simulink model "Controller_PP_test"  (R2021a)
settings: Solver=FixedStepDiscrete  StartTime=0.0  StopTime=inf  FixedStep=0.05  RelTol=1e-3
PostLoadFcn:
  | , if any(exist('dsrtsu_mdlpostloadfcn', 'file') == [2, 3, 6]), try dsrtsu_mdlpostloadfcn('Execute', bdroot); catch fprintf('Error in PostLoadFcn (dsrtsu_mdlpostloadfcn) for model "%s":\n %s\n', bdroot, lasterr); end, end,
model workspace (MAT data in the model file):
  DLC_kr = [-5.84862481044e-05 -6.43095507895e-05 -7.01328534794e-05 -7.5956156174e-05 -8.17794588731e-05 -8.76027615758e-05 -9.34260642811e-05 -9.92493669872e-05 -0.000105072669692 -0.000110895972393 -0.000116719275087 -0.000122542545808 ... (2080 elements, 1x2080)]
  DLC_thetar = [1.57172954906 1.57172588114 1.57172186534 1.57171750165 1.57171279008 1.57170773062 1.57170232328 1.57169656806 1.57169046495 1.57168401395 1.57167721507 1.57167006831 ... (2080 elements, 1x2080)]
  DLC_xr = [-0.00056695162723 -0.000622594591628 -0.000678008043004 -0.000733171198692 -0.000788063276025 -0.000842663492338 -0.000896951064963 -0.000950905211235 -0.00100450514849 -0.00105773009405 -0.00111055926527 -0.00116297187948 ... (2080 elements, 1x2080)]
  DLC_yr = [0.59999973213 0.659739817002 0.719479902091 0.779219987412 0.838960072984 0.898700158824 0.958440244948 1.01818033138 1.07792041812 1.1376605052 1.19740059264 1.25714068045 ... (2080 elements, 1x2080)]
  Fliter_ = 0.5
  Fliter_k = 1
  Iz = 1650
  SL_ROS_VariableLengthArrays_MaxSizes.CommonInfo.ArrayTruncateAction = 'EmitWarning'
  SL_ROS_VariableLengthArrays_MaxSizes.MsgTypeMap = containers.Map
  SL_ROS_VariableLengthArrays_MaxSizes.MsgTypeMap.serialization.keys = {'std_msgs/Float32MultiArray', 'std_msgs/Float64MultiArray', 'std_msgs/Int16MultiArray'}
  SL_ROS_VariableLengthArrays_MaxSizes.MsgTypeMap.serialization.values{1}.PropertyName = 'Data'
  SL_ROS_VariableLengthArrays_MaxSizes.MsgTypeMap.serialization.values{1}.DataType = 'single'
  SL_ROS_VariableLengthArrays_MaxSizes.MsgTypeMap.serialization.values{1}.MaxLength = 2004
  SL_ROS_VariableLengthArrays_MaxSizes.MsgTypeMap.serialization.values{2}.PropertyName = 'Data'
  SL_ROS_VariableLengthArrays_MaxSizes.MsgTypeMap.serialization.values{2}.DataType = 'double'
  SL_ROS_VariableLengthArrays_MaxSizes.MsgTypeMap.serialization.values{2}.MaxLength = 3
  SL_ROS_VariableLengthArrays_MaxSizes.MsgTypeMap.serialization.values{3}.PropertyName = 'Data'
  SL_ROS_VariableLengthArrays_MaxSizes.MsgTypeMap.serialization.values{3}.DataType = 'int16'
  SL_ROS_VariableLengthArrays_MaxSizes.MsgTypeMap.serialization.values{3}.MaxLength = 5
  SL_ROS_VariableLengthArrays_MaxSizes.MsgTypeMap.serialization.uniformity = 0
  SL_ROS_VariableLengthArrays_MaxSizes.MsgTypeMap.serialization.keyType = 'char'
  SL_ROS_VariableLengthArrays_MaxSizes.MsgTypeMap.serialization.valueType = 'any'
  a = 1
  b = 1.8
  cf = -120000
  cr = -120000
  factor_str = 0.15
  k1 = [0.258198889801 0.258198889749 0.258198889743 0.258198889805 0.258198889772 0.258198889764 0.258198889767 0.258198889768 0.258198889748 0.258198889747 0.258198889747 0.258198889747 ... (1000 elements, 1x1000)]
  k2 = [0.000225641086743 0.000451280556994 0.000676916794375 0.000902548182649 0.00112817310577 0.00135378994806 0.00157939709421 0.00180499292937 0.00203057583924 0.00225614421016 0.00248169642913 0.00270723088396 ... (1000 elements, 1x1000)]
  k3 = [1.8072435186 1.8072437178 1.80724404966 1.8072445143 1.80724511184 1.80724584231 1.80724670582 1.80724770248 1.80724883243 1.8072500958 1.80725149277 1.80725302351 ... (1000 elements, 1x1000)]
  k4 = [0.000229144738699 0.000458288056581 0.000687428532897 0.000916564747031 0.00114569527856 0.00137481870732 0.00160393361347 0.00183303857755 0.00206213218056 0.00229121300401 0.00252027963002 0.00274933064131 ... (1000 elements, 1x1000)]
  kr = [3.43040952456 5.20354947673 6.57526776383 5.89663744443 5.05963864905 4.19207203133 3.37422700169 2.64183787985 2.00068698258 1.44046440991 0.943931458435 0.491794250204 ... (89883 elements, 89883x1)]
  m = 1500
  straight_kr = [0 0 0 0 0 0 0 0 0 0 0 0 ... (10000 elements, 10000x1)]
  straight_thetar = [1.5708 1.5708 1.5708 1.5708 1.5708 1.5708 1.5708 1.5708 1.5708 1.5708 1.5708 1.5708 ... (10000 elements, 10000x1)]
  straight_xr = [0 0 0 0 0 0 0 0 0 0 0 0 ... (10000 elements, 10000x1)]
  straight_yr = [0.01 0.02 0.03 0.04 0.05 0.06 0.07 0.08 0.09 0.1 0.11 0.12 ... (10000 elements, 10000x1)]
  thetar = [0.0108871889919 0.137918447215 0.259619297152 0.371627288769 0.47112102891 0.556859678388 0.628810120477 0.687658443901 0.734398145371 0.77005371967 0.795522448239 0.811495552059 ... (89883 elements, 89883x1)]
  xr = [399944.786619 399944.805491 399944.823621 399944.841077 399944.857922 399944.874223 399944.890046 399944.905456 399944.920519 399944.935301 399944.949866 399944.964282 ... (89883 elements, 89883x1)]
  xr_init = 3407363.99438
  yr = [3406937.32043 3406937.32184 3406937.3255 3406937.33122 3406937.33879 3406937.34802 3406937.35871 3406937.37066 3406937.38366 3406937.39752 3406937.41203 3406937.427 ... (89883 elements, 89883x1)]
  yr_init = 400335.964759
undefined symbols (not defined in the file or in its folder): Data, Data_SL_Info
libraries: robotlib x5, simulink_extras x3
(part 1 of 2)
Description:
  | Standard RTI1401 template.
  | Supported MATLAB version:  R2018a.
settings Model: Tag=RTI1401  DSRTSU_INTERNAL_RTI_VER=520  DSRTSU_INTERNAL_RTI_TYPE=rti1401  RTICANMMDATA=struct('GeneralSetupData',struct('modelroot',['C:\Users\HS\Downloads\回复：LQR (1)'],'generalsettings',struct('filesettings',struct('destfolder',struct('Name','RTICANMM_FILES','Check',1),'buildfolder',struct('Name','.','Check',1),'AbsDestfolder',struct('Name',['C:\Users\HS\Downloads\回复：LQR (1)\RTICANMM_FILES']),'AbsBuildfolder',struct('Name',['C:\Users\HS\Downloads\回复：LQR (1)']))),'options',struct('addpaths',1,'rmpaths',1,'addtrcexclusion',logical(1),'cannavigator',struct('checkmonitoring',0),'show_usrtrc',0,'use_usrtrc',0),'advanced',struct('options',[1 1 1 1 1 1 1 1 1 1 1 1 1 1 1 1 1 1 1 1 1 1 1 1 1 1 1 1 1 1 1 1 1 1 1 1 1 1 1 1 1 1 1 1 1 1 1 1 1 1 1 1 1 1 1 1 1 1 1 1 1 1 1 1 1 1 1 1 1 1 1 1 1 1 1 1 1 1 1 1 1 1 1 1 1 1 1 1 1 1 1 1 1 1 1 1 1 1 1 1]),'MPSetup',{{}},'modelname','Path_Track_g','block','Path_Track_g'))  DSRTSU_INTERNAL_RTIFLEXRAYCONFIG=110  DSRTSU_INTERNAL_RTIFPGA=110  EnablePacing=on  OrderedModelArguments=off  Creator=HS  LastModifiedBy=xhu-fsac
settings SolverCC: AlgebraicLoopSolver=TrustRegion
settings DataIOCC: ReturnWorkspaceOutputs=off
settings OptimizationCC: BlockReduction=off  EnhancedBackFolding=on  PassReuseOutputArgsAs=Individual arguments  MaxStackSize=64  OptimizeBlockOrder=speed  DifferentSizesBufferReuse=on  OptimizationCustomize=off  EfficientTunableParamExpr=on
settings DebuggingCC: ParameterTunabilityLossMsg=error  PregeneratedLibrarySubsystemCodeDiagnostic=none  SFMachineParentedDataDiag=warning  ArithmeticOperatorsInVariantConditions=warning
settings HardwareCC: ProdBitPerPointer=32  ProdBitPerSizeT=32  ProdBitPerPtrDiffT=32  ProdLargestAtomicFloat=None  ProdIntDivRoundTo=Undefined  ProdEndianess=Unspecified  ProdWordSize=32  ProdHWDeviceType=Generic->Unspecified (assume 32-bit Generic)  TargetIntDivRoundTo=Zero  TargetEndianess=BigEndian  TargetHWDeviceType=Custom Processor->Custom
settings ModelReferenceCC: PropagateVarSize=During execution
settings SFSimCC: SimUseLocalCustomCode=off  CustomCodeUndefinedFunction=UseInterfaceOnly  SimTargetLang=C++
settings RTWCC: SystemTargetFile=ert.tlc  HardwareBoard=Robot Operating System (ROS)  TLCOptions="-aInlineSetEventsForThisBaseRateFcn=TLC_FALSE -aSuppressMultiTaskScheduler=TLC_FALSE  -aRateBasedStepFcn=0"  TemplateMakefile=ert_default_tmf  GenerateReport=on  RTWUseLocalCustomCode=off  Toolchain=Catkin  IncludeHyperlinkInReport=on  LaunchReport=on  TargetLang=C++  GenerateTraceInfo=on  GenerateTraceReport=on  GenerateTraceReportSl=on  GenerateTraceReportSf=on  GenerateTraceReportEml=on
settings CodeAppCC: ForceParamTrailComments=on  IgnoreCustomStorageClasses=off  OperatorAnnotations=on  SimulinkDataObjDesc=on  SFDataObjDesc=on  InsertBlockDesc=on
settings ERTTargetCC: SupportVariableSizeSignals=on
settings ConfigComp: CovMetricSettings=dswe

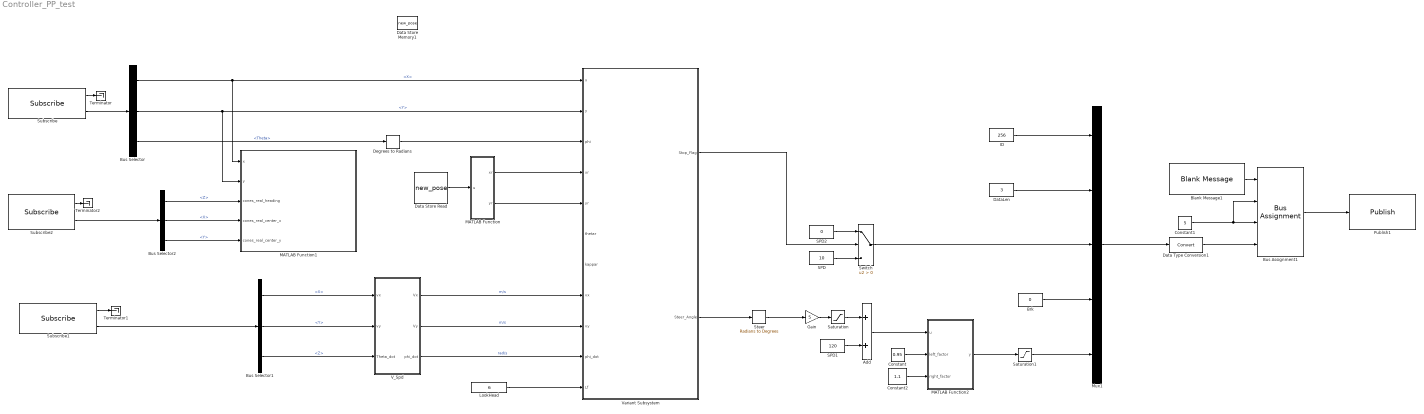
== system Controller_PP_test ==
  Add : Sum
  Blank Message1 : robotlib/Blank Message  messageClass=Message  entityType=std_msgs/Int16MultiArray  messageType=std_msgs/Int16MultiArray  SampleTime=-1  legacyBusStruct=off
  Brk : Constant  Value=0
  Bus Assignment1 : BusAssignment  AssignedSignals=Data_SL_Info.ReceivedLength,Data_SL_Info.CurrentLength,Data
  Bus Selector : BusSelector  OutputSignals=X,Y,Theta
  Bus Selector1 : BusSelector  OutputSignals=Linear.X,Linear.Y,Linear.Z
  Bus Selector2 : BusSelector  OutputSignals=Position.Z,Position.X,Position.Y
  Constant : Constant  Value=0.95
  Constant1 : Constant  Value=5  OutDataTypeStr=uint32  SampleTime=-1
  Constant2 : Constant  Value=1.1
  Data Store Memory1 : DataStoreMemory  DataStoreName=new_pose  ReadBeforeWriteMsg=warning  WriteAfterWriteMsg=warning  WriteAfterReadMsg=warning  ShowAdditionalParam=off  OutDataTypeStr=double  Dimensions=[191,2]
  Data Store Read : DataStoreRead  DataStoreName=new_pose  IndexOptions=Index vector (dialog)  Indices=1  OutputSizes=1
  Data Type Conversion1 : DataTypeConversion
  DataLen : Constant  Value=3
  Degrees to Radians : simulink_extras/Transformations/Degrees to Radians
  Gain : Gain  Gain=5
  ID : Constant  Value=256
  LookHead : Constant  Value=6
  MATLAB Function : MATLAB Function  TreatAsAtomicUnit=on
  MATLAB Function1 : MATLAB Function  TreatAsAtomicUnit=on
  MATLAB Function2 : MATLAB Function  TreatAsAtomicUnit=on
  Mux1 : Mux  Inputs=5
  Publish1 : robotlib/Publish  topicSource=Specify your own  topic=/send_can_msgs_port1  messageType=std_msgs/Int16MultiArray  legacyBusStruct=off  messageQueueLength=1
  SPD : Constant  Value=10
  SPD1 : Constant  Value=120
  SPD2 : Constant  Value=0
  Saturation : Saturate  UpperLimit=120  LowerLimit=-120
  Saturation1 : Saturate  UpperLimit=240  LowerLimit=0
  Steer : simulink_extras/Transformations/Radians to Degrees
  Subscribe : robotlib/Subscribe  topicSource=Specify your own  topic=/canalystii_ros/vehicle_Pose  messageType=geometry_msgs/Pose2D  SampleTime=0.05  legacyBusStruct=off  messageQueueLength=1
  Subscribe1 : robotlib/Subscribe  topicSource=Specify your own  topic=/canalystii_ros/vehicle_spd  messageType=geometry_msgs/Twist  SampleTime=0.05  legacyBusStruct=off  messageQueueLength=1
  Subscribe2 : robotlib/Subscribe  topicSource=Specify your own  topic=/point  messageType=geometry_msgs/Pose  SampleTime=-1  legacyBusStruct=off  messageQueueLength=1
  Switch : Switch  Criteria=u2 > Threshold
  Terminator : Terminator
  Terminator1 : Terminator
  Terminator2 : Terminator
  V_Spd : Subsystem
  Variant Subsystem : Subsystem  Variant=on  VariantControlMode=label  LabelModeActiveChoice=Controller == 5  AllowZeroVariantControls=on
  wires:
  V_Spd/3(phi_dot) -> Variant Subsystem/10(phi_dot)  "rad/s"
  Subscribe1/2 -> Bus Selector1/1
  Bus Selector1/3 -> V_Spd/3(Theta_dot)  "<Z>"
  V_Spd/1(Vx) -> Variant Subsystem/8(vx)  "m/s"
  Subscribe/2 -> Bus Selector/1
  Bus Selector/3 -> Degrees to Radians/1  "<Theta>"
  V_Spd/2(Vy) -> Variant Subsystem/9(vy)  "m/s"
  Subscribe/1 -> Terminator/1
  Subscribe1/1 -> Terminator1/1
  Bus Selector1/1 -> V_Spd/1(vx)  "<X>"
  Bus Selector1/2 -> V_Spd/2(vy)  "<Y>"
  Data Store Read/1 -> MATLAB Function/1(u)
  MATLAB Function/1(xr) -> Variant Subsystem/4(xr)
  MATLAB Function/2(yr) -> Variant Subsystem/5(yr)
  Brk/1 -> Mux1/4
  Saturation/1 -> Add/1
  Gain/1 -> Saturation/1
  Bus Assignment1/1 -> Publish1/1
  Steer/1 -> Gain/1
  Constant1/1 -> Bus Assignment1/2, Bus Assignment1/3
  ID/1 -> Mux1/1
  Variant Subsystem/2(Steer_Angle) -> Steer/1
  Mux1/1 -> Data Type Conversion1/1
  Data Type Conversion1/1 -> Bus Assignment1/4
  Blank Message1/1 -> Bus Assignment1/1
  SPD1/1 -> Add/2
  DataLen/1 -> Mux1/2
  Subscribe2/2 -> Bus Selector2/1
  Subscribe2/1 -> Terminator2/1
  Bus Selector/1 -> MATLAB Function1/1(x), Variant Subsystem/1(x)  "<X>"
  Degrees to Radians/1 -> Variant Subsystem/3(phi)
  Bus Selector2/1 -> MATLAB Function1/3(cones_real_heading)  "<Z>"
  Bus Selector/2 -> MATLAB Function1/2(y), Variant Subsystem/2(y)  "<Y>"
  Bus Selector2/2 -> MATLAB Function1/4(cones_real_center_x)  "<X>"
  Bus Selector2/3 -> MATLAB Function1/5(cones_real_center_y)  "<Y>"
  Variant Subsystem/1(Stop_Flag) -> Switch/2
  Switch/1 -> Mux1/3
  SPD/1 -> Switch/3
  SPD2/1 -> Switch/1
  LookHead/1 -> Variant Subsystem/11(Lf)
  Add/1 -> MATLAB Function2/1(u)
  MATLAB Function2/1(y) -> Saturation1/1
  Constant2/1 -> MATLAB Function2/3(right_factor)
  Constant/1 -> MATLAB Function2/2(left_factor)
  Saturation1/1 -> Mux1/5
